simulink library "SepehrMILLib"  (R2022a)
settings: Solver=VariableStepAuto  StartTime=0.0  StopTime=10.0  RelTol=1e-3
values from neighbouring files (symbols this model uses):
  visSampleTime = 0.1    [SPARCS_MIL_init.m]
undefined symbols (not defined in the file or in its folder): attitude, epoch, IAU, km, m, s, satellite, simulator, WMM2020
libraries: sharedtransform x14, aerolibconvert2 x11, aerolibutil x7, simulink_extras x5, vrlib x4, aerolibtransform2 x3, sharedutil x3, aerolibgravity2 x2, aerolibcelestial x2, aerolibobsolete x1, aerolibattitudesys x1, simulink x1
(part 1 of 2)
settings Model: Creator=AHKh  LastModifiedBy=AHKh

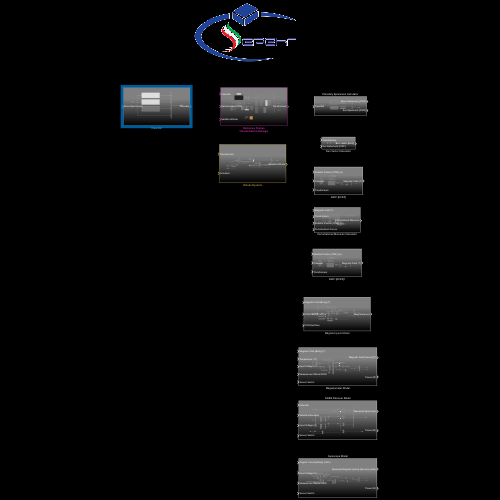
[thumbnail: Simulink's stored preview of the top-level diagram]
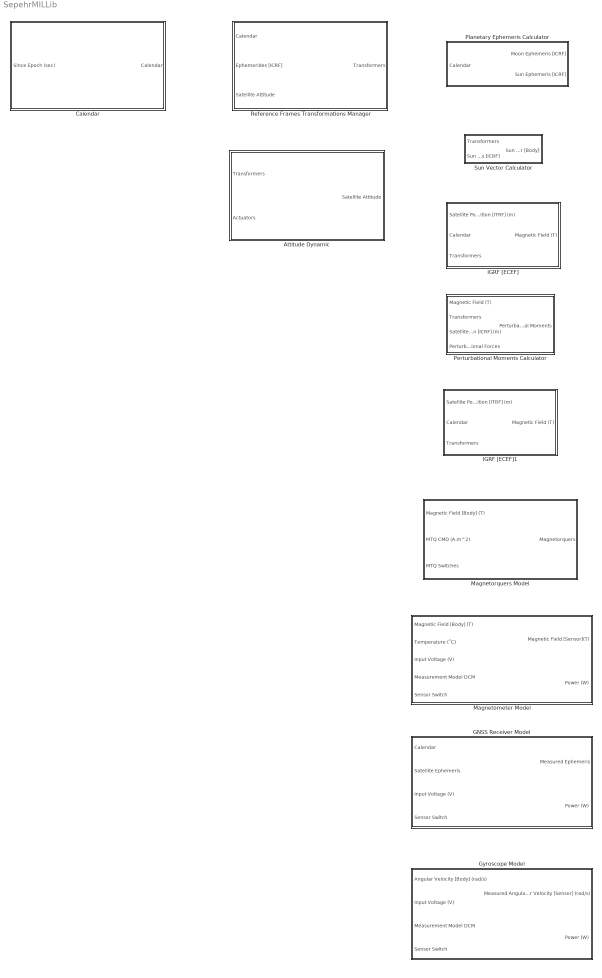
== system SepehrMILLib ==
  Attitude Dynamic : Subsystem
  Calendar : Subsystem
  GNSS Receiver Model : Subsystem
  Gyroscope Model : Subsystem
  IGRF [ECEF] : Subsystem
  IGRF [ECEF]1 : Subsystem
  Magnetometer Model : Subsystem
  Magnetorquers Model : Subsystem
  Perturbational Moments Calculator : Subsystem
  Planetary Ephemeris Calculator : Subsystem
  Reference Frames Transformations Manager : Subsystem
  Sun Vector Calculator : Subsystem

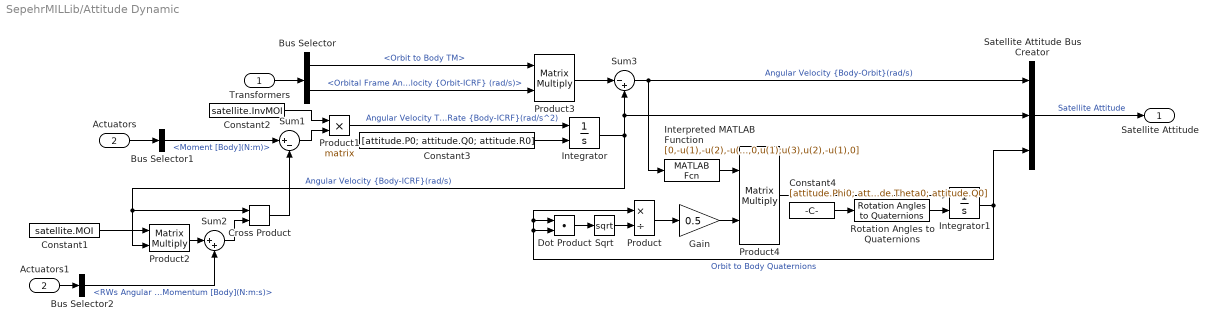
== system SepehrMILLib/Attitude Dynamic ==
  Transformers : Inport
  Actuators : Inport  Port=2
  Actuators1 : InportShadow  Port=2
  Bus Selector : BusSelector  OutputSignals=Transfer Matrices.Orbit to Body TM,Orbital Elements.Orbital Frame Angular Velocity {Orbit-ICRF} (rad/s)
  Bus Selector1 : BusSelector  OutputSignals=Momenta [Body].Moment [Body](N:m)
  Bus Selector2 : BusSelector  OutputSignals=Momenta [Body].RWs Angular Momentum [Body](N:m:s)
  Constant1 : Constant  Value=satellite.MOI
  Constant2 : Constant  Value=satellite.InvMOI
  Constant3 : Constant  Value=[attitude.P0; attitude.Q0; attitude.R0]
  Constant4 : Constant  Value=[attitude.Phi0; attitude.Theta0; attitude.Q0]
  Cross Product : vrlib/Utilities/Cross Product
  Dot Product : DotProduct  OutDataTypeStr=Inherit: Inherit via internal rule
  Gain : Gain  Gain=0.5
  Integrator : Integrator  InitialConditionSource=external  ContinuousStateAttributes={'P','Q','R'}
  Integrator1 : Integrator  InitialConditionSource=external  ContinuousStateAttributes={'q0','q1','q2','q3'}
  Interpreted MATLAB Function : MATLABFcn  MATLABFcn=[0,-u(1),-u(2),-u(3);u(1),0,u(3),-u(2);u(2),-u(3),0,u(1);u(3),u(2),-u(1),0]  OutputDimensions=[4,4]  OutputSignalType=real  Output1D=off
  Product : Product  Inputs=*/
  Product{1..4} (4 alike) : Product  Multiplication=Matrix(*)
  Rotation Angles to Quaternions : sharedtransform/Rotation Angles to Quaternions  rotationOrder=XYZ  aMode=aMode
      settings: SourceProductBaseCode=AE,PW,DR,MT,UV,VE
  Satellite Attitude Bus Creator : BusCreator  Inputs=3
  Sqrt : Sqrt  OutputSignalType=real
  Sum1 : Sum  Inputs=|+-
  Sum2 : Sum  Inputs=|++
  Sum3 : Sum  Inputs=|-+
  Satellite Attitude : Outport
  wires:
  Constant2/1 -> Product1/1
  Actuators/1 -> Bus Selector1/1
  Cross Product/1 -> Sum1/2
  Constant1/1 -> Product2/1
  Product2/1 -> Sum2/1
  Bus Selector2/1 -> Sum2/2  "<RWs Angular Momentum [Body](N:m:s)>"
  Sum2/1 -> Cross Product/2
  Sum1/1 -> Product1/2
  Product1/1 -> Integrator/1  "Angular Velocity Time Rate {Body-ICRF}(rad/s^2)"
  Transformers/1 -> Bus Selector/1
  Bus Selector/1 -> Product3/1  "<Orbit to Body TM>"
  Product3/1 -> Sum3/1
  Sum3/1 -> Interpreted MATLAB Function/1, Satellite Attitude Bus Creator/1  "Angular Velocity {Body-Orbit}(rad/s)"
  Constant3/1 -> Integrator/2
  Integrator/1 -> Sum3/2, Satellite Attitude Bus Creator/2, Product2/2, Cross Product/1  "Angular Velocity {Body-ICRF}(rad/s)"
  Dot Product/1 -> Sqrt/1
  Sqrt/1 -> Product/2
  Product/1 -> Gain/1
  Gain/1 -> Product4/2
  Interpreted MATLAB Function/1 -> Product4/1
  Product4/1 -> Integrator1/1
  Constant4/1 -> Rotation Angles to Quaternions/1
  Integrator1/1 -> Dot Product/1, Product/1, Dot Product/2, Satellite Attitude Bus Creator/3  "Orbit to Body Quaternions"
  Satellite Attitude Bus Creator/1 -> Satellite Attitude/1  "Satellite Attitude"
  Rotation Angles to Quaternions/1 -> Integrator1/2
  Bus Selector/2 -> Product3/2  "<Orbital Frame Angular Velocity {Orbit-ICRF} (rad/s)>"
  Bus Selector1/1 -> Sum1/1  "<Moment [Body](N:m)>"
  Actuators1/1 -> Bus Selector2/1

== system SepehrMILLib/Calendar ==
  Since Epoch (sec) : Inport  OutDataTypeStr=double  Unit=s  PortDimensions=1
  Calendar Bus Creator : BusCreator  Inputs=4
  Constant6 : Constant  Value=epoch.DecimalYear
  JD : Subsystem
  MJD : Subsystem
  Calendar : Outport
  wires:
  Since Epoch (sec)/1 -> JD/1(Since Epoch (sec)), Calendar Bus Creator/4, MJD/1(Since Epoch (sec))  "Since Epoch (sec)"
  JD/1(Julian Date (day)) -> Calendar Bus Creator/1  "Julian Date (day)"
  MJD/1(Modified Julian Date (day)) -> Calendar Bus Creator/2  "Modified Julian Date (day)"
  Constant6/1 -> Calendar Bus Creator/3  "Decimal Year (year)"
  Calendar Bus Creator/1 -> Calendar/1  "Calendar"

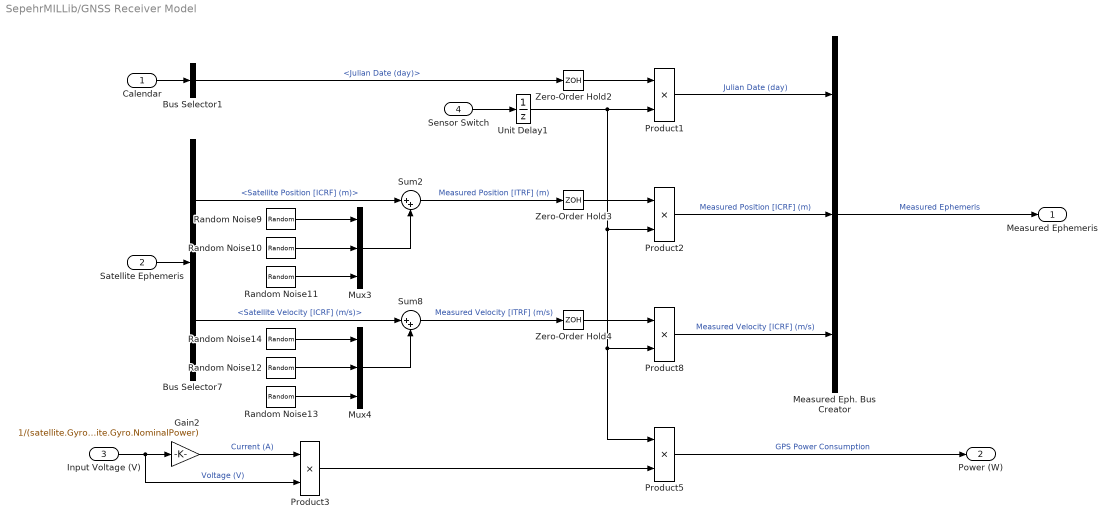
== system SepehrMILLib/GNSS Receiver Model ==
  Calendar : Inport
  Satellite Ephemeris : Inport  Port=2
  Input Voltage (V) : Inport  Port=3
  Sensor Switch : Inport  Port=4
  Bus Selector1 : BusSelector  OutputSignals=Julian Date (day)
  Bus Selector7 : BusSelector  OutputSignals=Satellite Position [ICRF] (m),Satellite Velocity [ICRF] (m/s)
  Gain2 : Gain  Gain=1/(satellite.Gyro.NominalVoltage^2/satellite.Gyro.NominalPower)
  Measured Eph. Bus Creator : BusCreator  Inputs=3
  Mux3 : Mux  Inputs=3
  Mux4 : Mux  Inputs=3
  Product{1..3,5,8} (5 alike) : Product
  Random Noise10 : RandomNumber  Mean=satellite.GPS.Position.Bias  Variance=satellite.GPS.Position.NoiseSTDDEV^2  SampleTime=1/satellite.GPS.Frequency
  Random Noise11 : RandomNumber  Mean=satellite.GPS.Position.Bias  Variance=satellite.GPS.Position.NoiseSTDDEV^2  SampleTime=1/satellite.GPS.Frequency
  Random Noise12 : RandomNumber  Mean=satellite.GPS.Velocity.Bias  Variance=satellite.GPS.Position.NoiseSTDDEV^2  SampleTime=1/satellite.GPS.Frequency
  Random Noise13 : RandomNumber  Mean=satellite.GPS.Velocity.Bias  Variance=satellite.GPS.Position.NoiseSTDDEV^2  SampleTime=1/satellite.GPS.Frequency
  Random Noise14 : RandomNumber  Mean=satellite.GPS.Velocity.Bias  Variance=satellite.GPS.Position.NoiseSTDDEV^2  SampleTime=1/satellite.GPS.Frequency
  Random Noise9 : RandomNumber  Mean=satellite.GPS.Position.Bias  Variance=satellite.GPS.Position.NoiseSTDDEV^2  SampleTime=1/satellite.GPS.Frequency
  Sum2 : Sum  Inputs=|++
  Sum8 : Sum  Inputs=|++
  Unit Delay1 : UnitDelay  SampleTime=-1  HasFrameUpgradeWarning=on
  Zero-Order Hold2 : ZeroOrderHold  SampleTime=1/satellite.GPS.Frequency
  Zero-Order Hold3 : ZeroOrderHold  SampleTime=1/satellite.GPS.Frequency
  Zero-Order Hold4 : ZeroOrderHold  SampleTime=1/satellite.GPS.Frequency
  Measured Ephemeris : Outport
  Power (W) : Outport  Port=2
  wires:
  Zero-Order Hold4/1 -> Product8/1
  Zero-Order Hold3/1 -> Product2/1
  Zero-Order Hold2/1 -> Product1/1
  Product8/1 -> Measured Eph. Bus Creator/3  "Measured Velocity [ICRF] (m/s)"
  Product2/1 -> Measured Eph. Bus Creator/2  "Measured Position [ICRF] (m)"
  Product1/1 -> Measured Eph. Bus Creator/1  "Julian Date (day)"
  Unit Delay1/1 -> Product1/2, Product2/2, Product8/2, Product5/1
  Sensor Switch/1 -> Unit Delay1/1
  Measured Eph. Bus Creator/1 -> Measured Ephemeris/1  "Measured Ephemeris"
  Bus Selector1/1 -> Zero-Order Hold2/1  "<Julian Date (day)>"
  Sum8/1 -> Zero-Order Hold4/1  "Measured Velocity [ITRF] (m/s)"
  Random Noise14/1 -> Mux4/1
  Random Noise13/1 -> Mux4/3
  Random Noise12/1 -> Mux4/2
  Mux4/1 -> Sum8/2
  Bus Selector7/2 -> Sum8/1  "<Satellite Velocity [ICRF] (m/s)>"
  Mux3/1 -> Sum2/2
  Random Noise10/1 -> Mux3/2
  Random Noise11/1 -> Mux3/3
  Random Noise9/1 -> Mux3/1
  Sum2/1 -> Zero-Order Hold3/1  "Measured Position [ITRF] (m)"
  Bus Selector7/1 -> Sum2/1  "<Satellite Position [ICRF] (m)>"
  Calendar/1 -> Bus Selector1/1
  Satellite Ephemeris/1 -> Bus Selector7/1
  Product5/1 -> Power (W)/1  "GPS Power Consumption"
  Input Voltage (V)/1 -> Gain2/1, Product3/2  "Voltage (V)"
  Gain2/1 -> Product3/1  "Current (A)"
  Product3/1 -> Product5/2

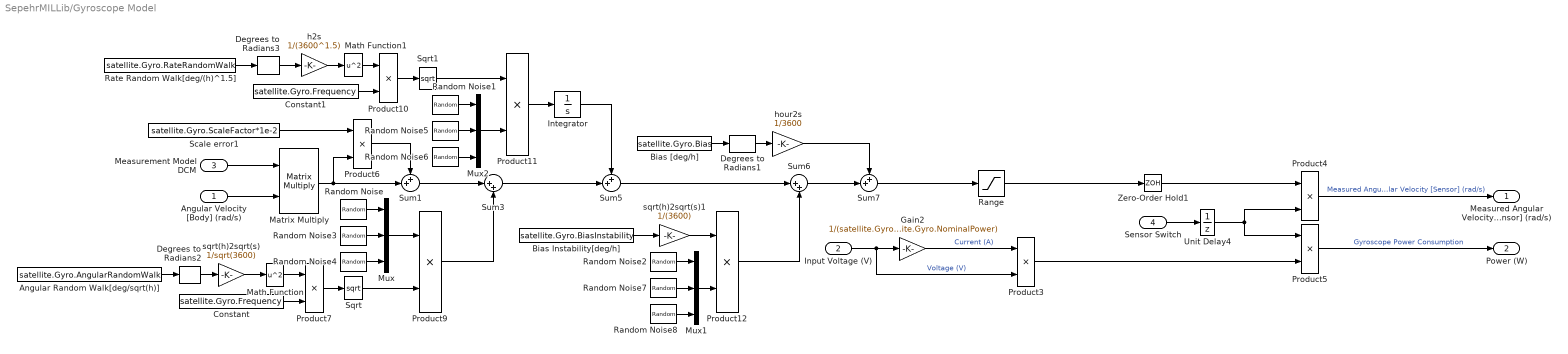
== system SepehrMILLib/Gyroscope Model ==
  Angular Velocity [Body] (rad/s) : Inport
  Input Voltage (V) : Inport  Port=2
  Measurement Model DCM : Inport  Port=3
  Sensor Switch : Inport  Port=4
  Angular Random Walk[deg/sqrt(h)] : Constant  Value=satellite.Gyro.AngularRandomWalk
  Bias Instability[deg/h] : Constant  Value=satellite.Gyro.BiasInstability
  Bias [deg/h] : Constant  Value=satellite.Gyro.Bias
  Constant : Constant  Value=satellite.Gyro.Frequency
  Constant1 : Constant  Value=satellite.Gyro.Frequency
  Degrees to Radians1 : simulink_extras/Transformations/Degrees to Radians
  Degrees to Radians2 : simulink_extras/Transformations/Degrees to Radians
  Degrees to Radians3 : simulink_extras/Transformations/Degrees to Radians
  Gain2 : Gain  Gain=1/(satellite.Gyro.NominalVoltage^2/satellite.Gyro.NominalPower)
  Integrator : Integrator  InitialCondition=[0;0;0]
  Math Function : Math  Operator=square  SignedPower=on
  Math Function1 : Math  Operator=square  SignedPower=on
  Matrix Multiply : Product  Multiplication=Matrix(*)
  Mux : Mux  Inputs=3
  Mux1 : Mux  Inputs=3
  Mux2 : Mux  Inputs=3
  Product{3..7,9..12} (9 alike) : Product
  Random Noise{,1..8} (9 alike) : RandomNumber  SampleTime=1/satellite.Gyro.Frequency
  Range : Saturate  UpperLimit=satellite.Gyro.Range(2)  LowerLimit=satellite.Gyro.Range(1)
  Rate Random Walk[deg/(h)^1.5] : Constant  Value=satellite.Gyro.RateRandomWalk
  Scale error1 : Constant  Value=satellite.Gyro.ScaleFactor*1e-2
  Sqrt : Sqrt
  Sqrt1 : Sqrt
  Sum1 : Sum  Inputs=++|
  Sum3 : Sum  Inputs=|++
  Sum5 : Sum  Inputs=++|
  Sum6 : Sum  Inputs=|++
  Sum7 : Sum  Inputs=++|
  Unit Delay4 : UnitDelay  SampleTime=-1  HasFrameUpgradeWarning=on
  Zero-Order Hold1 : ZeroOrderHold  SampleTime=1/satellite.Gyro.Frequency
  h2s : Gain  Gain=1/(3600^1.5)
  hour2s : Gain  Gain=1/3600
  sqrt(h)2sqrt(s) : Gain  Gain=1/sqrt(3600)
  sqrt(h)2sqrt(s)1 : Gain  Gain=1/(3600)
  Measured Angular Velocity [Sensor] (rad/s) : Outport  PortDimensions=[3,1]
  Power (W) : Outport  Port=2
  wires:
  Product5/1 -> Power (W)/1  "Gyroscope Power Consumption"
  Unit Delay4/1 -> Product5/1, Product4/2
  Product4/1 -> Measured Angular Velocity [Sensor] (rad/s)/1  "Measured Angular Velocity [Sensor] (rad/s)"
  Sensor Switch/1 -> Unit Delay4/1
  Zero-Order Hold1/1 -> Product4/1
  Measurement Model DCM/1 -> Matrix Multiply/1
  Angular Velocity [Body] (rad/s)/1 -> Matrix Multiply/2
  Input Voltage (V)/1 -> Product3/2, Gain2/1  "Voltage (V)"
  Gain2/1 -> Product3/1  "Current (A)"
  Product3/1 -> Product5/2
  Product10/1 -> Sqrt1/1
  Degrees to Radians3/1 -> h2s/1
  Degrees to Radians2/1 -> sqrt(h)2sqrt(s)/1
  Bias Instability[deg/h]/1 -> sqrt(h)2sqrt(s)1/1
  Bias [deg/h]/1 -> Degrees to Radians1/1
  Degrees to Radians1/1 -> hour2s/1
  sqrt(h)2sqrt(s)1/1 -> Product12/1
  Mux2/1 -> Product11/2
  Product11/1 -> Integrator/1
  Scale error1/1 -> Product6/1
  Mux/1 -> Product9/1
  Constant1/1 -> Product10/2
  Sqrt1/1 -> Product11/1
  Constant/1 -> Product7/2
  Rate Random Walk[deg/(h)^1.5]/1 -> Degrees to Radians3/1
  Math Function1/1 -> Product10/1
  Math Function/1 -> Product7/1
  sqrt(h)2sqrt(s)/1 -> Math Function/1
  Sqrt/1 -> Product9/2
  Product7/1 -> Sqrt/1
  Angular Random Walk[deg/sqrt(h)]/1 -> Degrees to Radians2/1
  Range/1 -> Zero-Order Hold1/1
  Sum7/1 -> Range/1
  h2s/1 -> Math Function1/1
  Matrix Multiply/1 -> Product6/2, Sum1/2
  Product6/1 -> Sum1/1
  Random Noise4/1 -> Mux/3
  Random Noise3/1 -> Mux/2
  Random Noise/1 -> Mux/1
  Product9/1 -> Sum3/2
  Sum1/1 -> Sum3/1
  Random Noise1/1 -> Mux2/1
  Random Noise6/1 -> Mux2/3
  Random Noise5/1 -> Mux2/2
  Random Noise2/1 -> Mux1/1
  Random Noise8/1 -> Mux1/3
  Random Noise7/1 -> Mux1/2
  Mux1/1 -> Product12/2
  Sum3/1 -> Sum5/2
  Integrator/1 -> Sum5/1
  Sum5/1 -> Sum6/1
  Product12/1 -> Sum6/2
  Sum6/1 -> Sum7/2
  hour2s/1 -> Sum7/1

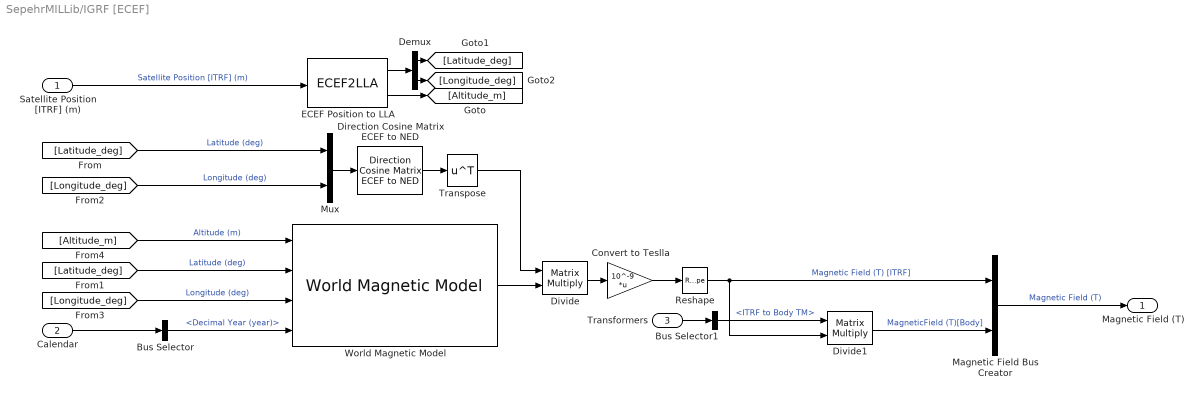
== system SepehrMILLib/IGRF [ECEF] ==
  Satellite Position [ITRF] (m) : Inport
  Calendar : Inport  Port=2
  Transformers : Inport  Port=3
  Bus Selector : BusSelector  OutputSignals=Decimal Year (year)
  Bus Selector1 : BusSelector  OutputSignals=Transfer Matrices.ITRF to Body TM
  Convert to Teslla : Gain  Gain=10^-9  Multiplication=Matrix(K*u)
  Demux : Demux  Outputs=2
  Direction Cosine Matrix ECEF to NED : aerolibtransform2/Direction Cosine Matrix ECEF to NED
      settings: SourceProductBaseCode=AE
  Divide : Product  Inputs=**  Multiplication=Matrix(*)
  Divide1 : Product  Inputs=**  Multiplication=Matrix(*)
  ECEF Position to LLA : ECEF2LLA
  Magnetic Field Bus Creator : BusCreator  Inputs=2
  Mux : Mux  Inputs=2
  Reshape : Reshape  OutputDimensionality=Customize  OutputDimensions=[3,1]
  Transpose : Math  Operator=transpose
  World Magnetic Model : aerolibgravity2/World Magnetic Model  model=WMM2020 (2020-2025)  customFile='WMM2020.COF'  units=Metric (MKS)  time_in=on  month=January  day=1  year=2020  action=Error  h_out=off  dec_out=off  inc_out=off  ti_out=off
      settings: SourceProductBaseCode=AE
  Magnetic Field (T) : Outport  OutDataTypeStr=double  Unit=T
  wires:
  Reshape/1 -> Divide1/2, Magnetic Field Bus Creator/1  "Magnetic Field (T) [ITRF]"
  Direction Cosine Matrix ECEF to NED/1 -> Transpose/1
  [Latitude_deg] -> World Magnetic Model/2  "Latitude (deg)"
  [Altitude_m] -> World Magnetic Model/1  "Altitude (m)"
  World Magnetic Model/1 -> Divide/2
  [Latitude_deg] -> Mux/1  "Latitude (deg)"
  [Longitude_deg] -> Mux/2  "Longitude (deg)"
  Divide/1 -> Convert to Teslla/1
  Calendar/1 -> Bus Selector/1
  Transpose/1 -> Divide/1
  Mux/1 -> Direction Cosine Matrix ECEF to NED/1
  [Longitude_deg] -> World Magnetic Model/3  "Longitude (deg)"
  Bus Selector/1 -> World Magnetic Model/4  "<Decimal Year (year)>"
  ECEF Position to LLA/1 -> Demux/1
  Demux/1 -> [Latitude_deg]
  Demux/2 -> [Longitude_deg]
  ECEF Position to LLA/2 -> [Altitude_m]
  Satellite Position [ITRF] (m)/1 -> ECEF Position to LLA/1  "Satellite Position [ITRF] (m)"
  Transformers/1 -> Bus Selector1/1
  Bus Selector1/1 -> Divide1/1  "<ITRF to Body TM>"
  Divide1/1 -> Magnetic Field Bus Creator/2  "MagneticField (T)[Body]"
  Magnetic Field Bus Creator/1 -> Magnetic Field (T)/1  "Magnetic Field (T)"
  Convert to Teslla/1 -> Reshape/1

== system SepehrMILLib/IGRF [ECEF]1 ==
  Satellite Position [ITRF] (m) : Inport
  Calendar : Inport  Port=2
  Transformers : Inport  Port=3
  Bus Selector : BusSelector  OutputSignals=Decimal Year (year)
  Bus Selector1 : BusSelector  OutputSignals=Transfer Matrices.ITRF to Body TM
  Convert to Teslla : Gain  Gain=10^-9  Multiplication=Matrix(K*u)
  Demux : Demux  Outputs=2
  Direction Cosine Matrix ECEF to NED : aerolibtransform2/Direction Cosine Matrix ECEF to NED
      settings: SourceProductBaseCode=AE
  Divide : Product  Inputs=**  Multiplication=Matrix(*)
  Divide1 : Product  Inputs=**  Multiplication=Matrix(*)
  ECEF Position to LLA : ECEF2LLA
  Magnetic Field Bus Creator : BusCreator  Inputs=2
  Mux : Mux  Inputs=2
  Reshape : Reshape  OutputDimensionality=Customize  OutputDimensions=[3,1]
  Transpose : Math  Operator=transpose
  World Magnetic Model : aerolibgravity2/World Magnetic Model  model=WMM2020 (2020-2025)  customFile='WMM2020.COF'  units=Metric (MKS)  time_in=on  month=January  day=1  year=2020  action=Error  h_out=off  dec_out=off  inc_out=off  ti_out=off
      settings: SourceProductBaseCode=AE
  Magnetic Field (T) : Outport  OutDataTypeStr=double  Unit=T
  wires:
  Reshape/1 -> Divide1/2, Magnetic Field Bus Creator/1  "Magnetic Field (T) [ITRF]"
  Direction Cosine Matrix ECEF to NED/1 -> Transpose/1
  [Latitude_deg] -> World Magnetic Model/2  "Latitude (deg)"
  [Altitude_m] -> World Magnetic Model/1  "Altitude (m)"
  World Magnetic Model/1 -> Divide/2
  [Latitude_deg] -> Mux/1  "Latitude (deg)"
  [Longitude_deg] -> Mux/2  "Longitude (deg)"
  Divide/1 -> Convert to Teslla/1
  Calendar/1 -> Bus Selector/1
  Transpose/1 -> Divide/1
  Mux/1 -> Direction Cosine Matrix ECEF to NED/1
  [Longitude_deg] -> World Magnetic Model/3  "Longitude (deg)"
  Bus Selector/1 -> World Magnetic Model/4  "<Decimal Year (year)>"
  ECEF Position to LLA/1 -> Demux/1
  Demux/1 -> [Latitude_deg]
  Demux/2 -> [Longitude_deg]
  ECEF Position to LLA/2 -> [Altitude_m]
  Satellite Position [ITRF] (m)/1 -> ECEF Position to LLA/1  "Satellite Position [ITRF] (m)"
  Transformers/1 -> Bus Selector1/1
  Bus Selector1/1 -> Divide1/1  "<ITRF to Body TM>"
  Divide1/1 -> Magnetic Field Bus Creator/2  "MagneticField (T)[Body]"
  Magnetic Field Bus Creator/1 -> Magnetic Field (T)/1  "Magnetic Field (T)"
  Convert to Teslla/1 -> Reshape/1

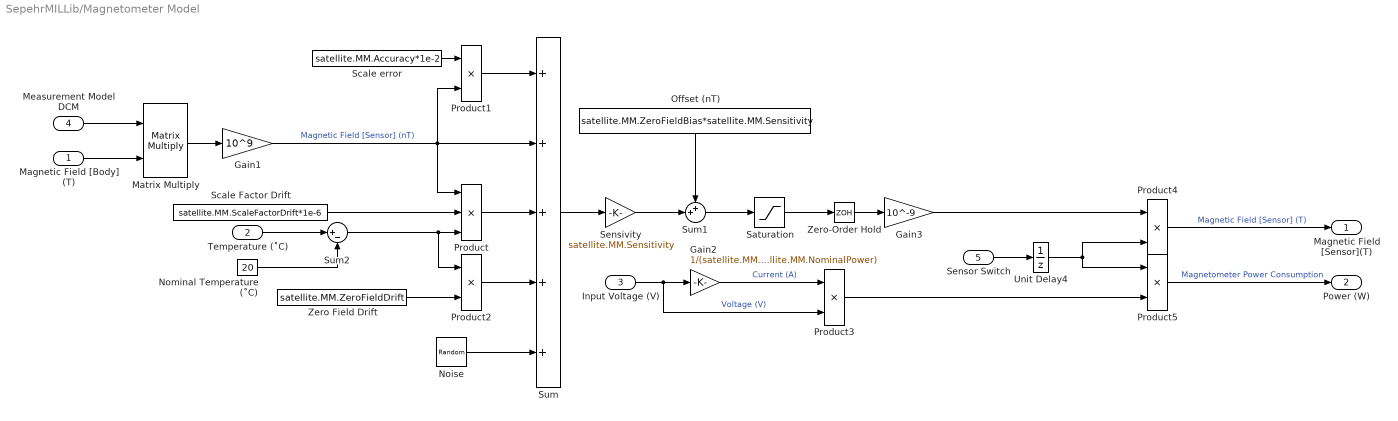
== system SepehrMILLib/Magnetometer Model ==
  Magnetic Field [Body] (T) : Inport
  Temperature (˚C) : Inport  Port=2
  Input Voltage (V) : Inport  Port=3
  Measurement Model DCM : Inport  Port=4
  Sensor Switch : Inport  Port=5
  Gain1 : Gain  Gain=10^9
  Gain2 : Gain  Gain=1/(satellite.MM.NominalVoltage^2/satellite.MM.NominalPower)
  Gain3 : Gain  Gain=10^-9
  Matrix Multiply : Product  Multiplication=Matrix(*)
  Noise : RandomNumber  Variance=satellite.MM.NoiseVariance  SampleTime=1/satellite.MM.Frequency
  Nominal Temperature (˚C) : Constant  Value=20
  Offset (nT) : Constant  Value=satellite.MM.ZeroFieldBias*satellite.MM.Sensitivity
  Product : Product  Inputs=3
  Product{1..5} (5 alike) : Product
  Saturation : Saturate  UpperLimit=satellite.MM.Range(2)  LowerLimit=satellite.MM.Range(1)
  Scale Factor Drift : Constant  Value=satellite.MM.ScaleFactorDrift*1e-6
  Scale error : Constant  Value=satellite.MM.Accuracy*1e-2
  Sensivity : Gain  Gain=satellite.MM.Sensitivity
  Sum : Sum  Inputs=+++++
  Sum1 : Sum  Inputs=++|
  Sum2 : Sum  Inputs=|+-
  Unit Delay4 : UnitDelay  SampleTime=-1  HasFrameUpgradeWarning=on
  Zero Field Drift : Constant  Value=satellite.MM.ZeroFieldDrift
  Zero-Order Hold : ZeroOrderHold  SampleTime=1/satellite.MM.Frequency
  Magnetic Field [Sensor](T) : Outport  PortDimensions=[3,1]
  Power (W) : Outport  Port=2
  wires:
  Offset (nT)/1 -> Sum1/1
  Sum/1 -> Sensivity/1
  Zero-Order Hold/1 -> Gain3/1
  Product3/1 -> Product5/2
  Gain2/1 -> Product3/1  "Current (A)"
  Input Voltage (V)/1 -> Gain2/1, Product3/2  "Voltage (V)"
  Saturation/1 -> Zero-Order Hold/1
  Product2/1 -> Sum/4
  Zero Field Drift/1 -> Product2/2
  Scale error/1 -> Product1/1
  Product1/1 -> Sum/1
  Scale Factor Drift/1 -> Product/2
  Sum2/1 -> Product/3, Product2/1
  Product/1 -> Sum/3
  Nominal Temperature (˚C)/1 -> Sum2/2
  Temperature (˚C)/1 -> Sum2/1
  Matrix Multiply/1 -> Gain1/1
  Sum1/1 -> Saturation/1
  Gain1/1 -> Product1/2, Product/1, Sum/2  "Magnetic Field [Sensor] (nT)"
  Magnetic Field [Body] (T)/1 -> Matrix Multiply/2
  Measurement Model DCM/1 -> Matrix Multiply/1
  Sensivity/1 -> Sum1/2
  Gain3/1 -> Product4/1
  Noise/1 -> Sum/5
  Sensor Switch/1 -> Unit Delay4/1
  Product4/1 -> Magnetic Field [Sensor](T)/1  "Magnetic Field [Sensor] (T)"
  Unit Delay4/1 -> Product4/2, Product5/1
  Product5/1 -> Power (W)/1  "Magnetometer Power Consumption"

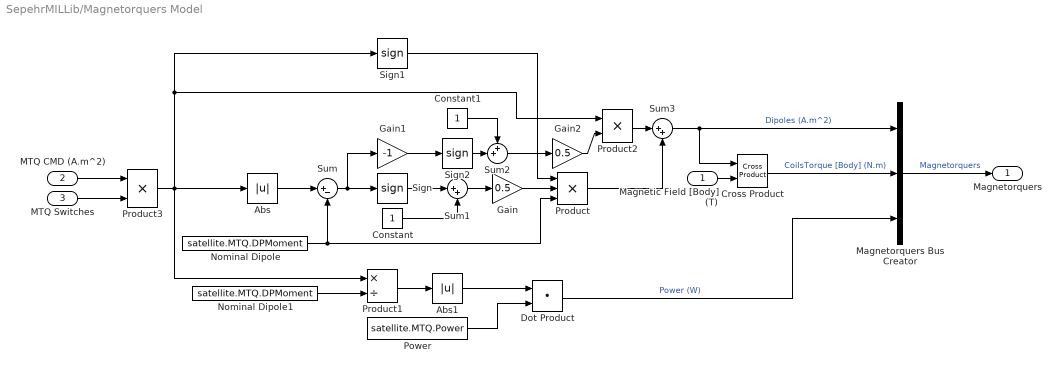
== system SepehrMILLib/Magnetorquers Model ==
  Magnetic Field [Body] (T) : Inport
  MTQ CMD (A.m^2) : Inport  Port=2  PortDimensions=[3,1]
  MTQ Switches : Inport  Port=3  PortDimensions=[3,1]
  Abs : Abs  SaturateOnIntegerOverflow=off
  Abs1 : Abs  SaturateOnIntegerOverflow=off
  Constant : Constant
  Constant1 : Constant
  Cross Product : vrlib/Utilities/Cross Product
  Dot Product : DotProduct  OutDataTypeStr=Inherit: Inherit via internal rule
  Gain : Gain  Gain=0.5
  Gain1 : Gain  Gain=-1
  Gain2 : Gain  Gain=0.5
  Magnetorquers Bus Creator : BusCreator  Inputs=3
  Nominal Dipole : Constant  Value=satellite.MTQ.DPMoment
  Nominal Dipole1 : Constant  Value=satellite.MTQ.DPMoment
  Power : Constant  Value=satellite.MTQ.Power
  Product : Product  Inputs=3
  Product1 : Product  Inputs=*/
  Product2 : Product
  Product3 : Product
  Sign : Signum
  Sign1 : Signum
  Sign2 : Signum
  Sum : Sum  Inputs=|+-
  Sum1 : Sum  Inputs=|++
  Sum2 : Sum  Inputs=++|
  Sum3 : Sum  Inputs=|++
  Magnetorquers : Outport
  wires:
  Product3/1 -> Abs/1, Product2/1, Sign1/1, Product1/1
  Nominal Dipole1/1 -> Product1/2
  Product1/1 -> Abs1/1
  Abs1/1 -> Dot Product/1
  Power/1 -> Dot Product/2
  Dot Product/1 -> Magnetorquers Bus Creator/3  "Power (W)"
  Product/1 -> Sum3/2
  Sum2/1 -> Gain2/1
  Magnetic Field [Body] (T)/1 -> Cross Product/2
  Gain1/1 -> Sign2/1
  Gain2/1 -> Product2/2
  Sum3/1 -> Cross Product/1, Magnetorquers Bus Creator/1  "Dipoles (A.m^2)"
  Product2/1 -> Sum3/1
  Constant/1 -> Sum1/2
  Sum1/1 -> Gain/1
  Cross Product/1 -> Magnetorquers Bus Creator/2  "CoilsTorque [Body] (N.m)"
  Sum/1 -> Gain1/1, Sign/1
  Constant1/1 -> Sum2/1
  Gain/1 -> Product/2
  Sign2/1 -> Sum2/2
  Sign1/1 -> Product/1
  Abs/1 -> Sum/1
  Nominal Dipole/1 -> Sum/2, Product/3
  Sign/1 -> Sum1/1
  MTQ CMD (A.m^2)/1 -> Product3/1
  MTQ Switches/1 -> Product3/2
  Magnetorquers Bus Creator/1 -> Magnetorquers/1  "Magnetorquers"

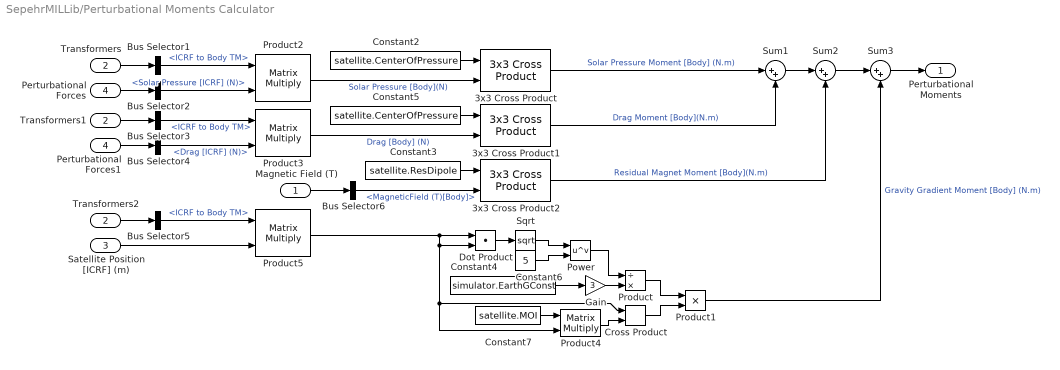
== system SepehrMILLib/Perturbational Moments Calculator ==
  Magnetic Field (T) : Inport
  Transformers : Inport  Port=2
  Satellite Position [ICRF] (m) : Inport  Port=3
  Perturbational Forces : Inport  Port=4
  3x3 Cross Product : sharedutil/3x3 Cross Product  aMode=aMode
      settings: SourceProductBaseCode=AE,PW,DR,MT,UV,VE
  3x3 Cross Product1 : sharedutil/3x3 Cross Product  aMode=aMode
      settings: SourceProductBaseCode=AE,PW,DR,MT,UV,VE
  3x3 Cross Product2 : sharedutil/3x3 Cross Product  aMode=aMode
      settings: SourceProductBaseCode=AE,PW,DR,MT,UV,VE
  Bus Selector1 : BusSelector  OutputSignals=Transfer Matrices.ICRF to Body TM
  Bus Selector2 : BusSelector  OutputSignals=|
      | Solar Pressure
      | [ICRF] (N)
  Bus Selector3 : BusSelector  OutputSignals=Transfer Matrices.ICRF to Body TM
  Bus Selector4 : BusSelector  OutputSignals=|
      | Drag
      | [ICRF] (N)
  Bus Selector5 : BusSelector  OutputSignals=Transfer Matrices.ICRF to Body TM
  Bus Selector6 : BusSelector  OutputSignals=|
      | MagneticField
      | (T)[Body]
  Constant2 : Constant  Value=satellite.CenterOfPressure
  Constant3 : Constant  Value=satellite.ResDipole
  Constant4 : Constant  Value=simulator.EarthGConst
  Constant5 : Constant  Value=satellite.CenterOfPressure
  Constant6 : Constant  Value=5
  Constant7 : Constant  Value=satellite.MOI
  Cross Product : vrlib/Utilities/Cross Product
  Dot Product : DotProduct  OutDataTypeStr=Inherit: Inherit via internal rule
  Gain : Gain  Gain=3
  Perturbational Forces1 : InportShadow  Port=4
  Power : Math  Operator=pow  OutputSignalType=real
  Product : Product  Inputs=/*
  Product1 : Product
  Product{2..5} (4 alike) : Product  Multiplication=Matrix(*)
  Sqrt : Sqrt  OutputSignalType=real
  Sum1 : Sum  Inputs=|++
  Sum2 : Sum  Inputs=|++
  Sum3 : Sum  Inputs=|++
  Transformers1 : InportShadow  Port=2
  Transformers2 : InportShadow  Port=2
  Perturbational Moments : Outport
  wires:
  3x3 Cross Product/1 -> Sum1/1  "Solar Pressure Moment [Body] (N.m)"
  Product2/1 -> 3x3 Cross Product/2  "Solar Pressure [Body](N)"
  3x3 Cross Product2/1 -> Sum2/2  "Residual Magnet Moment [Body](N.m)"
  3x3 Cross Product1/1 -> Sum1/2  "Drag Moment [Body](N.m)"
  Bus Selector5/1 -> Product5/1  "<ICRF to Body TM>"
  Product1/1 -> Sum3/2  "Gravity Gradient Moment [Body] (N.m)"
  Product3/1 -> 3x3 Cross Product1/2  "Drag [Body] (N)"
  Bus Selector3/1 -> Product3/1  "<ICRF to Body TM>"
  Transformers/1 -> Bus Selector1/1
  Bus Selector1/1 -> Product2/1  "<ICRF to Body TM>"
  Bus Selector2/1 -> Product2/2  "<Solar Pressure [ICRF] (N)>"
  Perturbational Forces/1 -> Bus Selector2/1
  Transformers1/1 -> Bus Selector3/1
  Bus Selector4/1 -> Product3/2  "<Drag [ICRF] (N)>"
  Perturbational Forces1/1 -> Bus Selector4/1
  Transformers2/1 -> Bus Selector5/1
  Satellite Position [ICRF] (m)/1 -> Product5/2
  Magnetic Field (T)/1 -> Bus Selector6/1
  Bus Selector6/1 -> 3x3 Cross Product2/2  "<MagneticField (T)[Body]>"
  Sum3/1 -> Perturbational Moments/1
  Constant2/1 -> 3x3 Cross Product/1
  Constant5/1 -> 3x3 Cross Product1/1
  Constant3/1 -> 3x3 Cross Product2/1
  Constant4/1 -> Gain/1
  Dot Product/1 -> Sqrt/1
  Product5/1 -> Product4/2, Cross Product/1, Dot Product/2, Dot Product/1
  Gain/1 -> Product/2
  Power/1 -> Product/1
  Sqrt/1 -> Power/1
  Constant6/1 -> Power/2
  Product/1 -> Product1/1
  Constant7/1 -> Product4/1
  Product4/1 -> Cross Product/2
  Cross Product/1 -> Product1/2
  Sum1/1 -> Sum2/1
  Sum2/1 -> Sum3/1

== system SepehrMILLib/Planetary Ephemeris Calculator ==
  Calendar : Inport
  Bus Selector : BusSelector  OutputSignals=Julian Date (day)
  Length Conversion : aerolibconvert2/Length Conversion  IU=km  OU=m
  Length Conversion1 : aerolibconvert2/Length Conversion  IU=km  OU=m
  Moon Ephemeris Bus Creator : BusCreator  Inputs=2
  Moon Ephemeris Calculator : aerolibcelestial/Planetary Ephemeris  kmflag=km,km/s  epochflag=Julian date  de=DE405  nCenter=Earth  nTarget=Moon  errorflag=Error  velflag=on
      settings: SourceProductBaseCode=AE
  Sun Ephemeris Bus Creator : BusCreator  Inputs=2
  Sun Ephemeris Calculator : aerolibcelestial/Planetary Ephemeris  kmflag=km,km/s  epochflag=Julian date  de=DE405  nCenter=Earth  nTarget=Sun  errorflag=Error  velflag=on
      settings: SourceProductBaseCode=AE
  Velocity Conversion : aerolibconvert2/Velocity Conversion  IU=km/s  OU=m/s
  Velocity Conversion1 : aerolibconvert2/Velocity Conversion  IU=km/s  OU=m/s
  Moon Ephemeris [ICRF] : Outport
  Sun Ephemeris [ICRF] : Outport  Port=2
  wires:
  Calendar/1 -> Bus Selector/1
  Bus Selector/1 -> Sun Ephemeris Calculator/1, Moon Ephemeris Calculator/1  "<Julian Date (day)>"
  Moon Ephemeris Calculator/1 -> Length Conversion/1
  Moon Ephemeris Calculator/2 -> Velocity Conversion/1
  Sun Ephemeris Calculator/2 -> Velocity Conversion1/1
  Sun Ephemeris Calculator/1 -> Length Conversion1/1
  Length Conversion/1 -> Moon Ephemeris Bus Creator/1  "Moon Position [ICRF] (m)"
  Velocity Conversion/1 -> Moon Ephemeris Bus Creator/2  "Moon Velocity [ICRF] (m/s)"
  Velocity Conversion1/1 -> Sun Ephemeris Bus Creator/2  "Sun Velocity [ICRF] (m/s)"
  Length Conversion1/1 -> Sun Ephemeris Bus Creator/1  "Sun Position [ICRF] (m)"
  Moon Ephemeris Bus Creator/1 -> Moon Ephemeris [ICRF]/1  "Moon Ephemeris [ICRF]"
  Sun Ephemeris Bus Creator/1 -> Sun Ephemeris [ICRF]/1  "Sun Ephemeris [ICRF]"

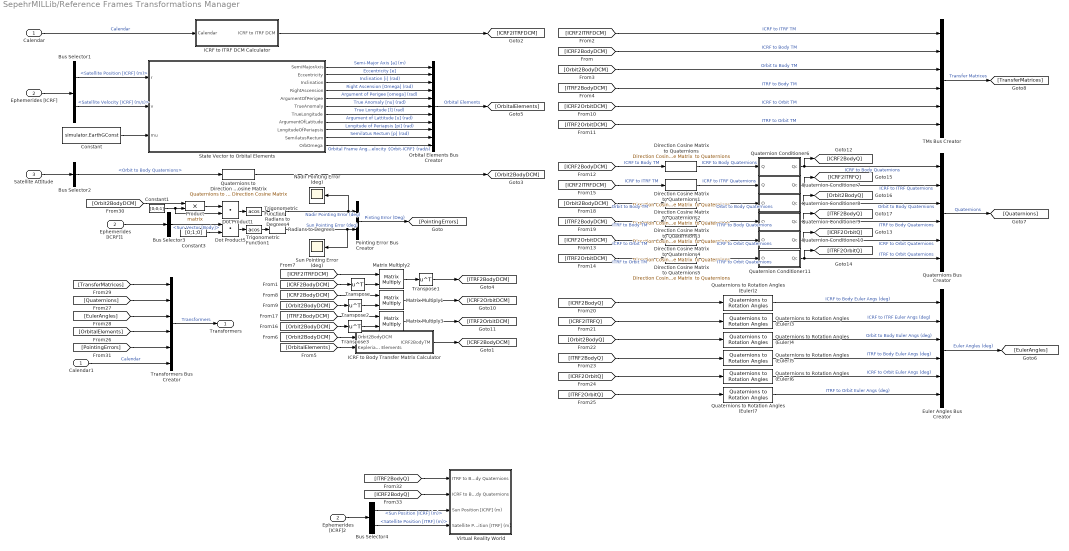
== system SepehrMILLib/Reference Frames Transformations Manager ==
  Calendar : Inport
  Ephemerides [ICRF] : Inport  Port=2
  Satellite Attitude : Inport  Port=3
  Bus Selector1 : BusSelector  OutputSignals=Satellite Ephemeris [ICRF].Satellite Position [ICRF] (m),Satellite Ephemeris [ICRF].Satellite Velocity [ICRF] (m/s)
  Bus Selector2 : BusSelector  OutputSignals=Orbit to Body Quaternions
  Bus Selector3 : BusSelector  OutputSignals=Satellite Ephemeris [ICRF].Sun Vector [Body]
  Bus Selector4 : BusSelector  OutputSignals=Sun Ephemeris [ICRF].Sun Position [ICRF] (m),Satellite Ephemeris [ICRF].Satellite Position [ITRF] (m)
  Calendar1 : InportShadow
  Constant : Constant  Value=simulator.EarthGConst
  Constant1 : Constant  Value=[0;0;1]
  Constant3 : Constant  Value=[0;1;0]
  Direction Cosine Matrix to Quaternions{,1..5} (6 alike) : sharedtransform/Direction Cosine Matrix  to Quaternions  aMode=0  action=None  tolerance=eps(2)
      settings: SourceProductBaseCode=AE,PW,DR,MT,UV,VE
  Dot Product1 : DotProduct  OutDataTypeStr=Inherit: Inherit via internal rule
  Dot Product5 : DotProduct  OutDataTypeStr=Inherit: Inherit via internal rule
  Ephemerides [ICRF]1 : InportShadow  Port=2
  Ephemerides [ICRF]2 : InportShadow  Port=2
  Euler Angles Bus Creator : BusCreator  Inputs=6
  ICRF to Body Transfer Matrix Calculator : Subsystem
  ICRF to ITRF DCM Calculator : Subsystem
  Matrix Multiply1 : Product  Multiplication=Matrix(*)
  Matrix Multiply2 : Product  Multiplication=Matrix(*)
  Matrix Multiply3 : Product  Multiplication=Matrix(*)
  Nadir Pointing Error (deg) : Scope
  Orbital Elements Bus Creator : BusCreator  Inputs=11
  Pointing Error Bus Creator : BusCreator  Inputs=2
  Product : Product  Multiplication=Matrix(*)
  Quaternion Conditioner10 : Subsystem
  Quaternion Conditioner11 : Subsystem
  Quaternion Conditioner6 : Subsystem
  Quaternion Conditioner7 : Subsystem
  Quaternion Conditioner8 : Subsystem
  Quaternion Conditioner9 : Subsystem
  Quaternions Bus Creator : BusCreator  Inputs=6
  Quaternions to Direction Cosine Matrix : sharedtransform/Quaternions to  Direction Cosine Matrix  aMode=aMode
      settings: SourceProductBaseCode=AE,PW,DR,MT,UV,VE
  Quaternions to Rotation Angles (Euler){2..7} (6 alike) : sharedtransform/Quaternions to Rotation Angles  rotationOrder=XYZ  aMode=aMode
      settings: SourceProductBaseCode=AE,PW,DR,MT,UV,VE
  Radians to Degrees : simulink_extras/Transformations/Radians to Degrees
  Radians to Degrees4 : simulink_extras/Transformations/Radians to Degrees
  State Vector to Orbital Elements : MATLAB Function  TreatAsAtomicUnit=on
  Sun Pointing Error (deg) : Scope
  TMs Bus Creator : BusCreator  Inputs=6
  Transformers Bus Creator : BusCreator  Inputs=6
  Transpose{,1..3} (4 alike) : Math  Operator=transpose
  Trigonometric Function : Trigonometry  Operator=acos
  Trigonometric Function1 : Trigonometry  Operator=acos  OutputSignalType=real
  Virtual Reality World : Subsystem  VariantControl=visSL3D
  Transformers : Outport
  wires:
  [ICRF2BodyDCM] -> TMs Bus Creator/2  "ICRF to Body TM"
  [ICRF2ITRFDCM] -> TMs Bus Creator/1  "ICRF to ITRF TM"
  [Orbit2BodyDCM] -> TMs Bus Creator/3  "Orbit to Body TM"
  [ITRF2BodyDCM] -> TMs Bus Creator/4  "ITRF to Body TM"
  [ICRF2OrbitDCM] -> TMs Bus Creator/5  "ICRF to Orbit TM"
  [ITRF2OrbitDCM] -> TMs Bus Creator/6  "ITRF to Orbit TM"
  TMs Bus Creator/1 -> [TransferMatrices]  "Transfer Matrices"
  Quaternions Bus Creator/1 -> [Quaternions]  "Quaternions"
  Direction Cosine Matrix to Quaternions5/1 -> Quaternion Conditioner11/1(Q)  "ITRF to Orbit Quaternions"
  Direction Cosine Matrix to Quaternions4/1 -> Quaternion Conditioner10/1(Q)  "ICRF to Orbit Quaternions"
  Direction Cosine Matrix to Quaternions3/1 -> Quaternion Conditioner9/1(Q)  "ITRF to Body Quaternions"
  Direction Cosine Matrix to Quaternions2/1 -> Quaternion Conditioner8/1(Q)  "Orbit to Body Quaternions"
  Direction Cosine Matrix to Quaternions1/1 -> Quaternion Conditioner7/1(Q)  "ICRF to ITRF Quaternions"
  Direction Cosine Matrix to Quaternions/1 -> Quaternion Conditioner6/1(Q)  "ICRF to Body Quaternions"
  Quaternions to Rotation Angles (Euler)2/1 -> Euler Angles Bus Creator/1  "ICRF to Body Euler Angs (deg)"
  Quaternions to Rotation Angles (Euler)3/1 -> Euler Angles Bus Creator/2  "ICRF to ITRF Euler Angs (deg)"
  Quaternions to Rotation Angles (Euler)4/1 -> Euler Angles Bus Creator/3  "Orbit to Body Euler Angs (deg)"
  Quaternions to Rotation Angles (Euler)5/1 -> Euler Angles Bus Creator/4  "ITRF to Body Euler Angs (deg)"
  Quaternions to Rotation Angles (Euler)6/1 -> Euler Angles Bus Creator/5  "ICRF to Orbit Euler Angs (deg)"
  Quaternions to Rotation Angles (Euler)7/1 -> Euler Angles Bus Creator/6  "ITRF to Orbit Euler Angs (deg)"
  Euler Angles Bus Creator/1 -> [EulerAngles]  "Euler Angles (deg)"
  [ICRF2BodyDCM] -> Direction Cosine Matrix to Quaternions/1  "ICRF to Body TM"
  [ICRF2ITRFDCM] -> Direction Cosine Matrix to Quaternions1/1  "ICRF to ITRF TM"
  [Orbit2BodyDCM] -> Direction Cosine Matrix to Quaternions2/1  "Orbit to Body TM"
  [ITRF2BodyDCM] -> Direction Cosine Matrix to Quaternions3/1  "ITRF to Body TM"
  [ICRF2OrbitDCM] -> Direction Cosine Matrix to Quaternions4/1  "ICRF to Orbit TM"
  [ITRF2OrbitDCM] -> Direction Cosine Matrix to Quaternions5/1  "ITRF to Orbit TM"
  [ICRF2BodyQ] -> Quaternions to Rotation Angles (Euler)2/1
  [ICRF2ITRFQ] -> Quaternions to Rotation Angles (Euler)3/1
  [Orbit2BodyQ] -> Quaternions to Rotation Angles (Euler)4/1
  [ITRF2BodyQ] -> Quaternions to Rotation Angles (Euler)5/1
  [ICRF2OrbitQ] -> Quaternions to Rotation Angles (Euler)6/1
  [ITRF2OrbitQ] -> Quaternions to Rotation Angles (Euler)7/1
  Quaternion Conditioner6/1(Qc) -> [ICRF2BodyQ], Quaternions Bus Creator/1  "ICRF to Body Quaternions"
  Quaternion Conditioner7/1(Qc) -> [ICRF2ITRFQ], Quaternions Bus Creator/2  "ICRF to ITRF Quaternions"
  Quaternion Conditioner8/1(Qc) -> [Orbit2BodyQ], Quaternions Bus Creator/3  "Orbit to Body Quaternions"
  Quaternion Conditioner9/1(Qc) -> [ITRF2BodyQ], Quaternions Bus Creator/4  "ITRF to Body Quaternions"
  Quaternion Conditioner10/1(Qc) -> [ICRF2OrbitQ], Quaternions Bus Creator/5  "ICRF to Orbit Quaternions"
  Quaternion Conditioner11/1(Qc) -> [ITRF2OrbitQ], Quaternions Bus Creator/6  "ITRF to Orbit Quaternions"
  ICRF to Body Transfer Matrix Calculator/1(ICRF2BodyTM) -> [ICRF2BodyDCM]
  State Vector to Orbital Elements/6(TrueAnomaly) -> Orbital Elements Bus Creator/6  "True Anomaly [nu] (rad)"
  State Vector to Orbital Elements/3(Inclination) -> Orbital Elements Bus Creator/3  "Inclination [i] (rad)"
  State Vector to Orbital Elements/7(TrueLongitude) -> Orbital Elements Bus Creator/7  "True Longitude [l] (rad)"
  State Vector to Orbital Elements/2(Eccentricity) -> Orbital Elements Bus Creator/2  "Eccentricity [e]"
  Constant/1 -> State Vector to Orbital Elements/3(mu)
  State Vector to Orbital Elements/4(RightAscension) -> Orbital Elements Bus Creator/4  "Right Ascension [Omega] (rad)"
  State Vector to Orbital Elements/9(LongitudeOfPeriapsis) -> Orbital Elements Bus Creator/9  "Longitude of Periapsis [pi] (rad)"
  State Vector to Orbital Elements/10(SemilatusRectum) -> Orbital Elements Bus Creator/10  "Semilatus Rectum [p] (rad)"
  State Vector to Orbital Elements/1(SemiMajorAxis) -> Orbital Elements Bus Creator/1  "Semi-Major Axis [a] (m)"
  State Vector to Orbital Elements/5(ArgumentOfPerigee) -> Orbital Elements Bus Creator/5  "Argument of Perigee [omega] (rad)"
  State Vector to Orbital Elements/8(ArgumentOfLatitude) -> Orbital Elements Bus Creator/8  "Argument of Lattitude [u] (rad)"
  Ephemerides [ICRF]/1 -> Bus Selector1/1
  Bus Selector1/2 -> State Vector to Orbital Elements/2(v)  "<Satellite Velocity [ICRF] (m/s)>"
  Bus Selector1/1 -> State Vector to Orbital Elements/1(r)  "<Satellite Position [ICRF] (m)>"
  Calendar/1 -> ICRF to ITRF DCM Calculator/1(Calendar)  "Calendar"
  [OrbitalElements] -> ICRF to Body Transfer Matrix Calculator/2(Keplerian Elements)
  Satellite Attitude/1 -> Bus Selector2/1
  Bus Selector2/1 -> Quaternions to Direction Cosine Matrix/1  "<Orbit to Body Quaternions>"
  Quaternions to Direction Cosine Matrix/1 -> [Orbit2BodyDCM]
  [Orbit2BodyDCM] -> ICRF to Body Transfer Matrix Calculator/1(Orbit2BodyDCM)
  Orbital Elements Bus Creator/1 -> [OrbitalElements]  "Orbital Elements"
  ICRF to ITRF DCM Calculator/1(ICRF to ITRF DCM) -> [ICRF2ITRFDCM]
  [ICRF2BodyDCM] -> Transpose/1
  Transpose/1 -> Matrix Multiply2/2
  [ICRF2ITRFDCM] -> Matrix Multiply2/1
  Matrix Multiply2/1 -> Transpose1/1
  Transpose1/1 -> [ITRF2BodyDCM]
  [Orbit2BodyDCM] -> Transpose2/1
  Matrix Multiply1/1 -> [ICRF2OrbitDCM]
  Transpose2/1 -> Matrix Multiply1/2
  [ICRF2BodyDCM] -> Matrix Multiply1/1
  Matrix Multiply3/1 -> [ITRF2OrbitDCM]
  [Orbit2BodyDCM] -> Transpose3/1
  Transpose3/1 -> Matrix Multiply3/2
  [ITRF2BodyDCM] -> Matrix Multiply3/1
  State Vector to Orbital Elements/11(OrbOmega) -> Orbital Elements Bus Creator/11  "Orbital Frame Angular Velocity {Orbit-ICRF} (rad/s)"
  [OrbitalElements] -> Transformers Bus Creator/4
  [EulerAngles] -> Transformers Bus Creator/3
  [Quaternions] -> Transformers Bus Creator/2
  Transformers Bus Creator/1 -> Transformers/1  "Transformers"
  [TransferMatrices] -> Transformers Bus Creator/1
  Trigonometric Function/1 -> Radians to Degrees4/1
  Product/1 -> Dot Product1/1
  Dot Product1/1 -> Trigonometric Function/1
  Radians to Degrees4/1 -> Nadir Pointing Error (deg)/1, Pointing Error Bus Creator/1  "Nadir Pointing Error (deg)"
  Constant1/1 -> Dot Product1/2, Product/2
  [Orbit2BodyDCM] -> Product/1
  Dot Product5/1 -> Trigonometric Function1/1
  Bus Selector3/1 -> Dot Product5/1  "<Sun Vector [Body]>"
  Radians to Degrees/1 -> Pointing Error Bus Creator/2, Sun Pointing Error (deg)/1  "Sun Pointing Error (deg)"
  Constant3/1 -> Dot Product5/2
  Trigonometric Function1/1 -> Radians to Degrees/1
  Ephemerides [ICRF]1/1 -> Bus Selector3/1
  Pointing Error Bus Creator/1 -> [PointingErrors]  "Pinting Error (Deg)"
  [PointingErrors] -> Transformers Bus Creator/5
  Calendar1/1 -> Transformers Bus Creator/6  "Calendar"
  [ITRF2BodyQ] -> Virtual Reality World/1(ITRF to Body Quaternions)
  [ICRF2BodyQ] -> Virtual Reality World/2(ICRF to Body Quaternions)
  Ephemerides [ICRF]2/1 -> Bus Selector4/1
  Bus Selector4/2 -> Virtual Reality World/4(Satellite Position [ITRF] (m))  "<Satellite Position [ITRF] (m)>"
  Bus Selector4/1 -> Virtual Reality World/3(Sun Position [ICRF] (m))  "<Sun Position [ICRF] (m)>"

== system SepehrMILLib/Sun Vector Calculator ==
  Transformers : Inport
  Sun Ephemeris [ICRF] : Inport  Port=2
  Bus Selector1 : BusSelector  OutputSignals=Transfer Matrices.ICRF to Body TM
  Bus Selector5 : BusSelector  OutputSignals=Sun Position [ICRF] (m)
  Matrix Multiply2 : Product  Multiplication=Matrix(*)
  Normalization2 : dspmathops/Normalization  NormType=2-norm  Bias=1e-10  NormOver=Each column  Dimension=1  roundingMode=Floor  overflowMode=off  accumDataTypeStr=Inherit: Same as product output  accumLastDataTypeStr=Inherit: Same as product output  outputDataTypeStr=Inherit: Same as product output  outputMin=[]  outputMax=[]  outputLastDataTypeStr=Inherit: Same as product output
  Sun Vector [Body] : Outport
  wires:
  Bus Selector1/1 -> Matrix Multiply2/1  "<ICRF to Body TM>"
  Matrix Multiply2/1 -> Normalization2/1  "Sun Position [Body] (m)"
  Sun Ephemeris [ICRF]/1 -> Bus Selector5/1
  Normalization2/1 -> Sun Vector [Body]/1  "Sun Vector [Body]"
  Bus Selector5/1 -> Matrix Multiply2/2  "<Sun Position [ICRF] (m)>"
  Transformers/1 -> Bus Selector1/1

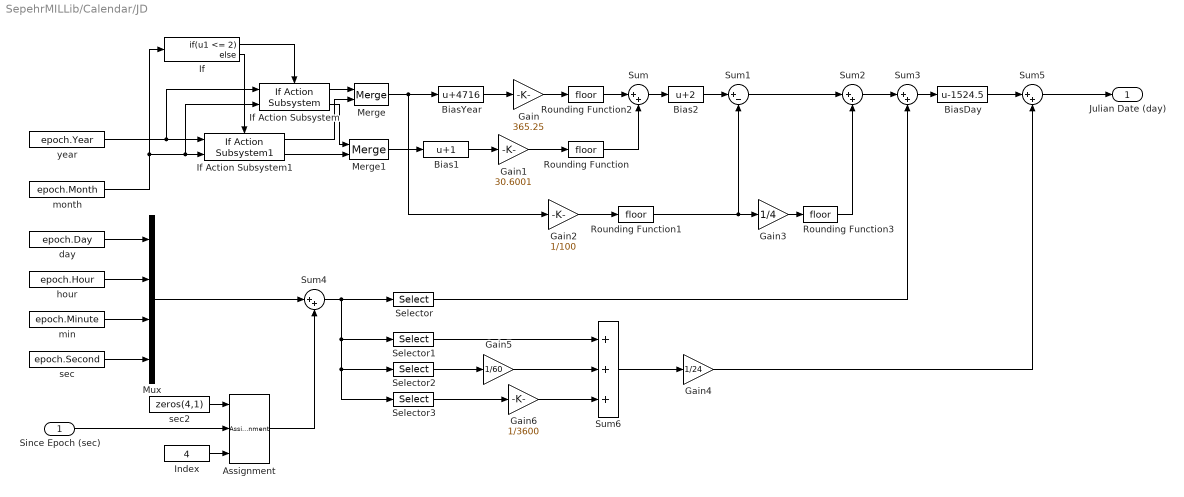
== system SepehrMILLib/Calendar/JD ==
  Since Epoch (sec) : Inport  OutMin=0  PortDimensions=1
  Assignment : Assignment  IndexOptions=Index vector (port)  Indices=1  OutputSizes=1
  Bias1 : Bias  Bias=1  SaturateOnIntegerOverflow=off
  Bias2 : Bias  Bias=2  SaturateOnIntegerOverflow=off
  BiasDay : Bias  Bias=-1524.5  SaturateOnIntegerOverflow=off
  BiasYear : Bias  Bias=4716  SaturateOnIntegerOverflow=off
  Gain : Gain  Gain=365.25
  Gain1 : Gain  Gain=30.6001
  Gain2 : Gain  Gain=1/100
  Gain3 : Gain  Gain=1/4
  Gain4 : Gain  Gain=1/24
  Gain5 : Gain  Gain=1/60
  Gain6 : Gain  Gain=1/3600
  If : If  IfExpression=u1 <= 2
  If Action Subsystem : aerolibconvert2/Julian Date Conversion/If Action Subsystem  SystemSampleTime=-1  VariantActivationTime=update diagram  Latency=0  AutoFrameSizeCalculation=off
      settings: SourceProductBaseCode=AE
  If Action Subsystem1 : aerolibconvert2/Julian Date Conversion/If Action Subsystem1  SystemSampleTime=-1  VariantActivationTime=update diagram  Latency=0  AutoFrameSizeCalculation=off
      settings: SourceProductBaseCode=AE
  Index : Constant  Value=4
  Merge : Merge
  Merge1 : Merge
  Mux : Mux
  Rounding Function{,1..3} (4 alike) : Rounding
  Selector : Selector  InputPortWidth=4  IndexOptions=Index vector (dialog)  Indices=[1]  OutputSizes=1
  Selector1 : Selector  InputPortWidth=4  IndexOptions=Index vector (dialog)  Indices=[2]  OutputSizes=1
  Selector2 : Selector  InputPortWidth=4  IndexOptions=Index vector (dialog)  Indices=[3]  OutputSizes=1
  Selector3 : Selector  InputPortWidth=4  IndexOptions=Index vector (dialog)  Indices=[4]  OutputSizes=1
  Sum{,2..5} (5 alike) : Sum  Inputs=|++
  Sum1 : Sum  Inputs=|+-
  Sum6 : Sum  Inputs=+++
  day : Constant  Value=epoch.Day
  hour : Constant  Value=epoch.Hour
  min : Constant  Value=epoch.Minute
  month : Constant  Value=epoch.Month
  sec : Constant  Value=epoch.Second
  sec2 : Constant  Value=zeros(4,1)
  year : Constant  Value=epoch.Year
  Julian Date (day) : Outport  VectorParamsAs1DForOutWhenUnconnected=off
  wires:
  Mux/1 -> Sum4/1
  Gain4/1 -> Sum5/2
  If/2 -> If Action Subsystem1/Action
  Selector1/1 -> Sum6/1
  Sum/1 -> Bias2/1
  Rounding Function3/1 -> Sum2/2
  Sum4/1 -> Selector1/1, Selector2/1, Selector3/1, Selector/1
  Assignment/1 -> Sum4/2
  Sum5/1 -> Julian Date (day)/1
  sec2/1 -> Assignment/1
  hour/1 -> Mux/2
  BiasDay/1 -> Sum5/1
  Sum6/1 -> Gain4/1
  Selector/1 -> Sum3/2
  Rounding Function2/1 -> Sum/1
  Gain5/1 -> Sum6/2
  Bias2/1 -> Sum1/1
  Gain/1 -> Rounding Function2/1
  Bias1/1 -> Gain1/1
  Gain3/1 -> Rounding Function3/1
  Gain6/1 -> Sum6/3
  Gain2/1 -> Rounding Function1/1
  Rounding Function1/1 -> Gain3/1, Sum1/2
  Since Epoch (sec)/1 -> Assignment/2
  Merge1/1 -> Bias1/1
  Sum1/1 -> Sum2/1
  BiasYear/1 -> Gain/1
  Sum3/1 -> BiasDay/1
  Sum2/1 -> Sum3/1
  Gain1/1 -> Rounding Function/1
  day/1 -> Mux/1
  Rounding Function/1 -> Sum/2
  year/1 -> If Action Subsystem/1, If Action Subsystem1/1
  If/1 -> If Action Subsystem/Action
  Selector2/1 -> Gain5/1
  Merge/1 -> Gain2/1, BiasYear/1
  If Action Subsystem1/1 -> Merge/2
  min/1 -> Mux/3
  Selector3/1 -> Gain6/1
  If Action Subsystem/1 -> Merge/1
  If Action Subsystem1/2 -> Merge1/2
  month/1 -> If Action Subsystem/2, If Action Subsystem1/2, If/1
  sec/1 -> Mux/4
  Index/1 -> Assignment/3
  If Action Subsystem/2 -> Merge1/1

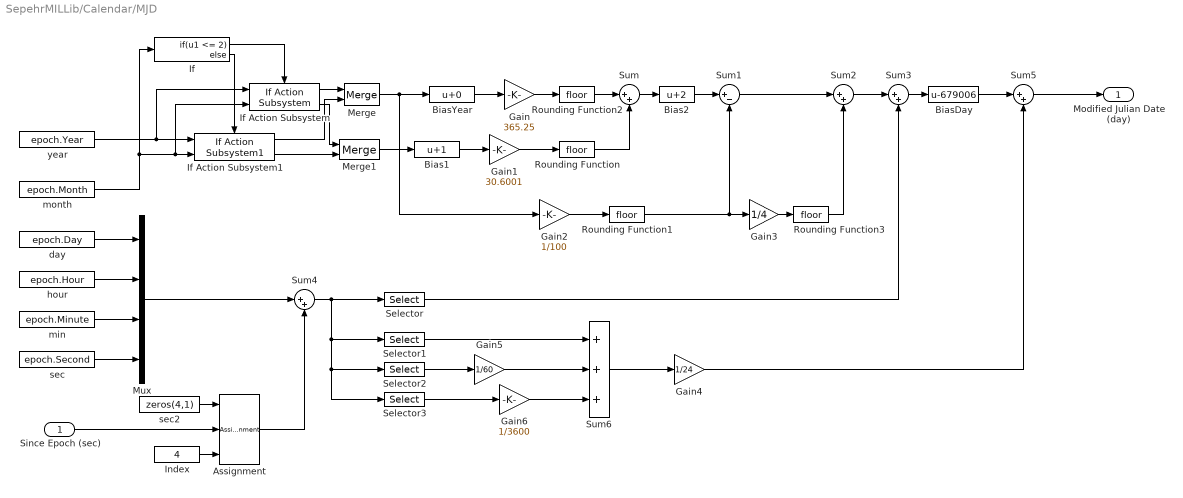
== system SepehrMILLib/Calendar/MJD ==
  Since Epoch (sec) : Inport  OutMin=0  PortDimensions=1
  Assignment : Assignment  IndexOptions=Index vector (port)  Indices=1  OutputSizes=1
  Bias1 : Bias  Bias=1  SaturateOnIntegerOverflow=off
  Bias2 : Bias  Bias=2  SaturateOnIntegerOverflow=off
  BiasDay : Bias  Bias=-679006  SaturateOnIntegerOverflow=off
  BiasYear : Bias  SaturateOnIntegerOverflow=off
  Gain : Gain  Gain=365.25
  Gain1 : Gain  Gain=30.6001
  Gain2 : Gain  Gain=1/100
  Gain3 : Gain  Gain=1/4
  Gain4 : Gain  Gain=1/24
  Gain5 : Gain  Gain=1/60
  Gain6 : Gain  Gain=1/3600
  If : If  IfExpression=u1 <= 2
  If Action Subsystem : aerolibconvert2/Julian Date Conversion/If Action Subsystem  SystemSampleTime=-1  VariantActivationTime=update diagram  Latency=0  AutoFrameSizeCalculation=off
      settings: SourceProductBaseCode=AE
  If Action Subsystem1 : aerolibconvert2/Julian Date Conversion/If Action Subsystem1  SystemSampleTime=-1  VariantActivationTime=update diagram  Latency=0  AutoFrameSizeCalculation=off
      settings: SourceProductBaseCode=AE
  Index : Constant  Value=4
  Merge : Merge
  Merge1 : Merge
  Mux : Mux
  Rounding Function{,1..3} (4 alike) : Rounding
  Selector : Selector  InputPortWidth=4  IndexOptions=Index vector (dialog)  Indices=[1]  OutputSizes=1
  Selector1 : Selector  InputPortWidth=4  IndexOptions=Index vector (dialog)  Indices=[2]  OutputSizes=1
  Selector2 : Selector  InputPortWidth=4  IndexOptions=Index vector (dialog)  Indices=[3]  OutputSizes=1
  Selector3 : Selector  InputPortWidth=4  IndexOptions=Index vector (dialog)  Indices=[4]  OutputSizes=1
  Sum{,2..5} (5 alike) : Sum  Inputs=|++
  Sum1 : Sum  Inputs=|+-
  Sum6 : Sum  Inputs=+++
  day : Constant  Value=epoch.Day
  hour : Constant  Value=epoch.Hour
  min : Constant  Value=epoch.Minute
  month : Constant  Value=epoch.Month
  sec : Constant  Value=epoch.Second
  sec2 : Constant  Value=zeros(4,1)
  year : Constant  Value=epoch.Year
  Modified Julian Date (day) : Outport  VectorParamsAs1DForOutWhenUnconnected=off
  wires:
  Mux/1 -> Sum4/1
  Gain4/1 -> Sum5/2
  If/2 -> If Action Subsystem1/Action
  Selector1/1 -> Sum6/1
  Sum/1 -> Bias2/1
  Rounding Function3/1 -> Sum2/2
  Sum4/1 -> Selector1/1, Selector2/1, Selector3/1, Selector/1
  Assignment/1 -> Sum4/2
  Sum5/1 -> Modified Julian Date (day)/1
  sec2/1 -> Assignment/1
  hour/1 -> Mux/2
  BiasDay/1 -> Sum5/1
  Sum6/1 -> Gain4/1
  Selector/1 -> Sum3/2
  Rounding Function2/1 -> Sum/1
  Gain5/1 -> Sum6/2
  Bias2/1 -> Sum1/1
  Gain/1 -> Rounding Function2/1
  Bias1/1 -> Gain1/1
  Gain3/1 -> Rounding Function3/1
  Gain6/1 -> Sum6/3
  Gain2/1 -> Rounding Function1/1
  Rounding Function1/1 -> Gain3/1, Sum1/2
  Since Epoch (sec)/1 -> Assignment/2
  Merge1/1 -> Bias1/1
  Sum1/1 -> Sum2/1
  BiasYear/1 -> Gain/1
  Sum3/1 -> BiasDay/1
  Sum2/1 -> Sum3/1
  Gain1/1 -> Rounding Function/1
  day/1 -> Mux/1
  Rounding Function/1 -> Sum/2
  year/1 -> If Action Subsystem/1, If Action Subsystem1/1
  If/1 -> If Action Subsystem/Action
  Selector2/1 -> Gain5/1
  Merge/1 -> Gain2/1, BiasYear/1
  If Action Subsystem1/1 -> Merge/2
  min/1 -> Mux/3
  Selector3/1 -> Gain6/1
  If Action Subsystem/1 -> Merge/1
  If Action Subsystem1/2 -> Merge1/2
  month/1 -> If Action Subsystem/2, If Action Subsystem1/2, If/1
  sec/1 -> Mux/4
  Index/1 -> Assignment/3
  If Action Subsystem/2 -> Merge1/1

== system SepehrMILLib/Reference Frames Transformations Manager/ICRF to Body Transfer Matrix Calculator ==
  Orbit2BodyDCM : Inport
  Keplerian Elements : Inport  Port=2
  Bus Selector : BusSelector  OutputSignals=Inclination [i] (rad),Right Ascension [Omega] (rad),Argument of Perigee [omega] (rad),True Anomaly [nu] (rad)
  Interpreted MATLAB Function : MATLABFcn  MATLABFcn=[cos(u),sin(u),0; -sin(u),cos(u),0; 0,0,1]  OutputDimensions=[3,3]  Output1D=off
  Interpreted MATLAB Function1 : MATLABFcn  MATLABFcn=[1,0,0;0,cos(u),sin(u);0,-sin(u),cos(u)]  OutputDimensions=[3,3]  Output1D=off
  Interpreted MATLAB Function2 : MATLABFcn  MATLABFcn=[cos(u),sin(u),0;-sin(u),cos(u),0;0,0,1]  OutputDimensions=[3,3]  Output1D=off
  Matrix Multiply{,1..3} (4 alike) : Product  Multiplication=Matrix(*)
  RotMat : Constant  Value=[0,1,0;0,0,-1;-1,0,0]
  Sum : Sum  Inputs=|++
  ICRF2BodyTM : Outport
  wires:
  Keplerian Elements/1 -> Bus Selector/1
  Bus Selector/1 -> Interpreted MATLAB Function1/1  "<Inclination [i] (rad)>"
  Bus Selector/2 -> Interpreted MATLAB Function2/1  "<Right Ascension [Omega] (rad)>"
  Bus Selector/3 -> Sum/1  "<Argument of Perigee [omega] (rad)>"
  Bus Selector/4 -> Sum/2  "<True Anomaly [nu] (rad)>"
  Sum/1 -> Interpreted MATLAB Function/1
  Interpreted MATLAB Function/1 -> Matrix Multiply/1
  Interpreted MATLAB Function1/1 -> Matrix Multiply/2
  Matrix Multiply/1 -> Matrix Multiply1/1
  Interpreted MATLAB Function2/1 -> Matrix Multiply1/2
  RotMat/1 -> Matrix Multiply2/1
  Matrix Multiply1/1 -> Matrix Multiply2/2
  Matrix Multiply2/1 -> Matrix Multiply3/2
  Orbit2BodyDCM/1 -> Matrix Multiply3/1
  Matrix Multiply3/1 -> ICRF2BodyTM/1

== system SepehrMILLib/Reference Frames Transformations Manager/ICRF to ITRF DCM Calculator ==
  note: **********************************************************************
      | * *
      | * I E R S B U L L E T I N - A *
      | * *
      | * Rapid Service/Prediction of Earth Orientation *
      | **********************************************************************
      | 30 September 2021 Vol. XXXIV No. 039
      | ______________________________________________________________________
      | GENERAL INFORMATION:
      | To receive this information electronically, contact:
      | ser7@maia.usno.navy.mil or use
      | <http://maia.usno.navy.mil/docrequest.html>
      | MJD = Julian Date - 2 400 000.5 days
      | UT2-UT1 = 0.022 sin(2*pi*T) - 0.012 cos(2*pi*T)
      | - 0.006 sin(4*pi*T) + 0.007 cos(4*pi*T)
      | where pi = 3.14159265... and T is the date in Besselian years.
      | TT = TAI + 32.184 seconds
      | DUT1= (UT1-UTC) transmitted with time signals
      | = -0.1 seconds beginning 17 July 2021 at 0000 UTC
      | Beginning 1 January 2017:
      | TAI-UTC = 37.000 000 seconds
  Calendar : Inport
  Bus Selector : BusSelector  OutputSignals=Modified Julian Date (day),Since Epoch (sec)
  Constant1 : Constant  Value=37
  Direction Cosine Matrix ICRF to ITRF : aerolibtransform2/Direction Cosine Matrix ECI to ECEF  red=IAU-2000/2006  year=2021  month=January  day=1  hour=12  min=0  sec=0  deltaT=Sec  errorflag=Error  extraparamflag=on
      settings: AttributesFormatString=%<red>  SourceProductBaseCode=AE
  Earth Orientation Parameters : EOParameters  FileName=aeroiersdata20211007.mat  iersurl=https://datacenter.iers.org/data/latestVersion/10_FINALS.DATA_IAU2000_V2013_0110.txt  folder=E:\A.H.Kh\My Current Projects\30-SepehrCube\SimpleMIL\ModelsData
  ICRF to ITRF DCM : Outport
  wires:
  Bus Selector/2 -> Direction Cosine Matrix ICRF to ITRF/5  "<Since Epoch (sec)>"
  Bus Selector/1 -> Earth Orientation Parameters/1  "<Modified Julian Date (day)>"
  Calendar/1 -> Bus Selector/1
  Direction Cosine Matrix ICRF to ITRF/1 -> ICRF to ITRF DCM/1
  Earth Orientation Parameters/2 -> Direction Cosine Matrix ICRF to ITRF/3  "Polar Displacement of Earth"
  Constant1/1 -> Direction Cosine Matrix ICRF to ITRF/2
  Earth Orientation Parameters/3 -> Direction Cosine Matrix ICRF to ITRF/4  "Celestial Intermediate Pole (CIP) Adjustment (radians)"
  Earth Orientation Parameters/1 -> Direction Cosine Matrix ICRF to ITRF/1

== system SepehrMILLib/Reference Frames Transformations Manager/Quaternion Conditioner10 ==
  Q : Inport  PortDimensions=[4,1]
  Interpreted MATLAB Function : MATLABFcn  MATLABFcn=[u(1),0,0,0;0,u(2),0,0;0,0,u(3),0;0,0,0,u(4)]
  Interpreted MATLAB Function1 : MATLABFcn  MATLABFcn=[u(1),0,0,0;0,u(2),0,0;0,0,u(3),0;0,0,0,u(4)]
  Interpreted MATLAB Function2 : MATLABFcn  MATLABFcn=(u(1)+u(6)+u(11)+u(16))+1.9
  Product : Product
  Product1 : Product
  Sign : Signum
  Sign1 : Signum
  Unit Delay : UnitDelay  InitialCondition=[1;0;0;0]  SampleTime=-1  HasFrameUpgradeWarning=on
  Qc : Outport  PortDimensions=[4,1]
  wires:
  Q/1 -> Interpreted MATLAB Function/1, Product1/1
  Unit Delay/1 -> Interpreted MATLAB Function1/1
  Sign1/1 -> Product1/2
  Interpreted MATLAB Function1/1 -> Product/2
  Sign/1 -> Interpreted MATLAB Function2/1
  Product/1 -> Sign/1
  Interpreted MATLAB Function/1 -> Product/1
  Product1/1 -> Qc/1, Unit Delay/1
  Interpreted MATLAB Function2/1 -> Sign1/1
